simulink model "squareWaveHarmonicsAnalysis"  (R2021a)
settings: Solver=VariableStepAuto  StartTime=0.0  StopTime=.04  FixedStep=.0001  MaxStep=.00001  RelTol=1e-3
InitFcn:
  | Freq=50;
libraries: spsFourierLib x1, spspowerguiLib x1
settings Model: Creator=User  LastModifiedBy=User

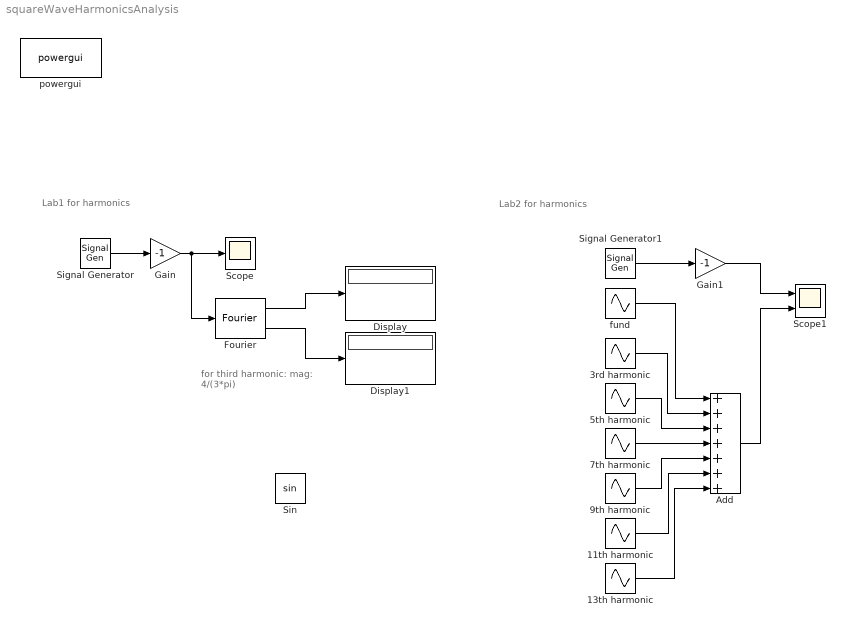
== system squareWaveHarmonicsAnalysis ==
  note: Lab2 for harmonics
  note: Lab1 for harmonics
  note: for third harmonic:
      | mag: 4/(3*pi)
  11th harmonic : Sin  Amplitude=4/(pi*11)  Frequency=Freq*11*(pi*2)  SampleTime=0
  13th harmonic : Sin  Amplitude=4/(pi*13)  Frequency=Freq*13*(pi*2)  SampleTime=0
  3rd harmonic : Sin  Amplitude=4/(pi*3)  Frequency=Freq*3*(pi*2)  SampleTime=0
  5th harmonic : Sin  Amplitude=4/(pi*5)  Frequency=Freq*5*(pi*2)  SampleTime=0
  7th harmonic : Sin  Amplitude=4/(pi*7)  Frequency=Freq*7*(pi*2)  SampleTime=0
  9th harmonic : Sin  Amplitude=4/(pi*9)  Frequency=Freq*9*(pi*2)  SampleTime=0
  Add : Sum  Inputs=+++++++
  Display : Display
  Display1 : Display
  Fourier : spsFourierLib/Fourier  Freq=50  n=3  InInit=[1, 0]  Ts=0
      settings: SourceProductBaseCode=PS
  Gain : Gain  Gain=-1
  Gain1 : Gain  Gain=-1
  Scope : Scope
  Scope1 : Scope  NumInputPorts=2
  Signal Generator : SignalGenerator  WaveForm=square  Frequency=50
  Signal Generator1 : SignalGenerator  WaveForm=square  Frequency=Freq
  Sin : Trigonometry
  fund : Sin  Amplitude=4/(pi*1)  Frequency=Freq*(pi*2)  SampleTime=0
  powergui : spspowerguiLib/powergui  Priority=1  SimulationMode=Discrete  SampleTime=50e-6  frequency=60  Iterations=50  frequencyindice=60  Pbase=100e6  ErrMax=1e-4  UnitsV=kV  UnitsW=MW  buscounter=0  FunctionMessages=off  echomessages=off  EnableUseOfTLC=off  CurrentSourceSwitches=off  DisableSnubberDevices=off  DisableRonSwitches=off  DisableVfSwitches=off  DisplayEquations=off  AutomaticDiscreteSolvers=off  SolverType=Tustin/Backward Euler (TBE)  Interpol=off  ExternalGateDelay=off  methode=off  Ts=100  x0status=blocks  SPID=on  SwTol=0  HookPort=off  NonlinearTolerance=1e-4  nMaxIteration=100  ContinueOnMaxIteration=off  RestoreLinks=warning  ResistiveCurrentMeasurement=off  Frange=[0:2:500]  Ylog=off  Xlog=on  ShowGrid=off  save=off  variable=ZData  structure=0  ZoomFFT=off  StartTime=0.0  cycles=1  DisplayStyle=1  fundamental=60  FreqAxis=off  MaxFrequency=1000  frequencyindicesteady=1  RmsSteady=1  display=off
  wires:
  Signal Generator/1 -> Gain/1
  Gain/1 -> Fourier/1, Scope/1
  Fourier/1 -> Display/1
  Fourier/2 -> Display1/1
  Signal Generator1/1 -> Gain1/1
  fund/1 -> Add/1
  3rd harmonic/1 -> Add/2
  5th harmonic/1 -> Add/3
  7th harmonic/1 -> Add/4
  Add/1 -> Scope1/2
  Gain1/1 -> Scope1/1
  9th harmonic/1 -> Add/5
  11th harmonic/1 -> Add/6
  13th harmonic/1 -> Add/7
